simulink model "PenduloSimple"  (R2024b)
settings: Solver=ode4  StartTime=0.0  StopTime=15.0  FixedStep=0.01  RelTol=1e-3
model workspace (MATLAB code in the model file):
  | x0 = -2*pi:0.1:2*pi;
settings Model: Creator=Miguel  LastModifiedBy=Miguel

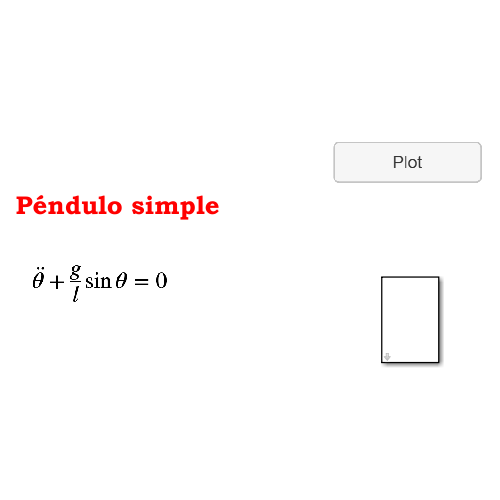
[thumbnail: Simulink's stored preview of the top-level diagram]
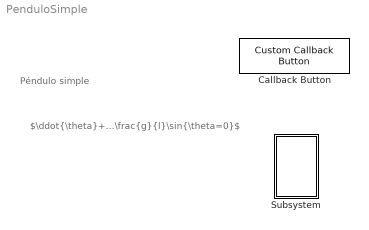
== system PenduloSimple ==
  note: $\ddot{\theta}+\frac{g}{l}\sin{\theta=0}$
  note: Péndulo simple
  Callback Button : CustomCallbackButton  Configuration="{\"components\":[{\"name\":\"BackgroundImageComponent\",\"settings\":{\"image\":{\"size\":[0,0],\"src\":\"default\",\"srcOrientation\":\"Right\"},\"position\":[0,0,1,1]}},{\"name\":\"ButtonStateComponent\",\"settings\":{\"buttonType\":\"momentary\",\"clickFcn\":\"close all\\n\\nx = out.theta;\\ny = out.theta_dot;\\n\\nn = length(x(1,:));\\n\\nplot(x(:,2),y(:,2),'LineWidth',3)\\nhold on\\n\\nfor i=3:n\\n    plot(x(:,i),y(:,i),'LineWidth',3)\\nend\\n\\nxf = linspace(-3*pi,3*pi,2000);\\nyf = zeros(1,2000);\\nplot(xf,yf,'k--','LineWidth',2)\\n\\nxlim([-3*pi,3*pi])\\ngrid on\\nhold off\",\"onValue\":1,\"position\":[0,0,1,1],\"pressDelay\":\"500\",\"pressFcn\":\"\",\"repeatInterval\":\"0\",\"states\":[{\"horizontalAlignment\":\"center\",\"image\":{\"position\":[0,0,1,1],\"size\":[1,1],\"src\":\"default\",\"srcOrientation\":\"Right\"},\"label\":{\"color\":[0.01176470588,0.01176470588,0.01176470588,1],\"icon\":{\"size\":[0,0],\"src\":\"default\",\"srcOrientation\":\"Right\"},\"iconOffset\":0,\"iconPlacement\":\"left\",\"opacity\":1,\"show\":true,\"text\":{\"content\":\"Plot\",\"font\":\"Helvetica\"}},\"labelOffset\":[0,0],\"verticalAlignment\":\"middle\"},{\"horizontalAlignment\":\"center\",\"image\":{\"position\":[0,0,1,1],\"size\":[1,1],\"src\":\"default\",\"srcOrientation\":\"Right\"},\"label\":{\"color\":[0.01176470588,0.01176470588,0.01176470588,1],\"icon\":{\"size\":[0,0],\"src\":\"default\",\"srcOrientation\":\"Right\"},\"iconOffset\":0,\"iconPlacement\":\"left\",\"opacity\":1,\"show\":true,\"text\":{\"content\":\"Plot\",\"font\":\"Helvetica\"}},\"labelOffset\":[0,0],\"verticalAlignment\":\"middle\"},{\"horizontalAlignment\":\"center\",\"image\":{\"position\":[0,0,1,1],\"size\":[1,1],\"src\":\"default\",\"srcOrientation\":\"Right\"},\"label\":{\"color\":[0.01176470588,0.01176470588,0.01176470588,1],\"icon\":{\"size\":[0,0],\"src\":\"default\",\"srcOrientation\":\"Right\"},\"iconOffset\":0,\"iconPlacement\":\"left\",\"opacity\":1,\"show\":true,\"text\":{\"content\":\"Plot\",\"font\":\"Helvetica\"}},\"labelOffset\":[0,0],\"verticalAlignment\":\"middle\"},{\"horizontalAlignment\":\"center\",\"image\":{\"position\":[0,0,1,1],\"size\":[1,1],\"src\":\"default\",\"srcOrientation\":\"Right\"},\"label\":{\"color\":[0.01176470588,0.01176470588,0.01176470588,1],\"icon\":{\"size\":[0,0],\"src\":\"default\",\"srcOrientation\":\"Right\"},\"iconOffset\":0,\"iconPlacement\":\"left\",\"opacity\":1,\"show\":true,\"text\":{\"content\":\"Plot\",\"font\":\"Helvetica\"}},\"labelOffset\":[0,0],\"verticalAlignment\":\"middle\"}]}},{\"name\":\"ForegroundImageComponent\",\"settings\":{\"image\":{\"size\":[0,0],\"src\":\"default\",\"srcOrientation\":\"Right\"},\"isForeground\":1,\"position\":[0,0,1,1]}}],\"settings\":{\"BindingType\":\"standalone\",\"backgroundColor\":[244,244,244,1],\"backgroundOffset\":0.2,\"backgroundOpacity\":1,\"fixedAspectRatio\":\"off\",\"foregroundColor\":[0.01176470588,0.01176470588,0.01176470588,1],\"migratedFromLegacy\":true,\"useBackgroundColor\":true,\"variant\":\"callback\",\"version\":\"R2023a\"},\"type\":\"Button\"}"  CustomBackgroundColor="{\"color\":[0.9568627451,0.9568627451,0.9568627451],\"show\":true}"
  Subsystem : Subsystem  mask{g=9.8, l=9.8}
      mask prompts: g "Constante gravedad"; l "Longitud péndulo"

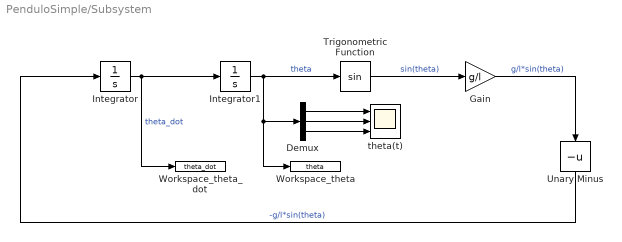
== system PenduloSimple/Subsystem ==
  Demux : Demux  Outputs=3
  Gain : Gain  Gain=g/l
  Integrator : Integrator
  Integrator1 : Integrator  InitialCondition=x0
  Trigonometric Function : Trigonometry
  Unary Minus : UnaryMinus
  Workspace_theta : ToWorkspace  VariableName=theta  SampleTime=-1
  Workspace_theta_dot : ToWorkspace  VariableName=theta_dot  SampleTime=-1
  theta(t) : Scope  NumInputPorts=3
  wires:
  Gain/1 -> Unary Minus/1  "g/l*sin(theta)"
  Trigonometric Function/1 -> Gain/1  "sin(theta)"
  Integrator/1 -> Workspace_theta_dot/1, Integrator1/1  "theta_dot"
  Unary Minus/1 -> Integrator/1  "-g/l*sin(theta)"
  Integrator1/1 -> Demux/1, Workspace_theta/1, Trigonometric Function/1  "theta"
  Demux/1 -> theta(t)/1
  Demux/2 -> theta(t)/2
  Demux/3 -> theta(t)/3
